simulink model "Sullivan_HodgkinHuxleyFinal"  (R2017a)
settings: Solver=ode45  StartTime=0.0  StopTime=100  RelTol=1e-3  EnableMultiTasking=on
settings Model: Creator=Andrew  LastModifiedBy=atsullivan
settings DataIOCC: LimitDataPoints=on  SaveFormat=Array
settings OptimizationCC: LifeSpan=inf
settings DebuggingCC: SFUnexpectedBacktrackingDiag=warning  SFNoUnconditionalDefaultTransitionDiag=warning  SFExecutionAtInitializationDiag=none
settings HardwareCC: ProdBitPerPointer=32  ProdBitPerSizeT=32  ProdBitPerPtrDiffT=32  ProdLargestAtomicFloat=None  ProdIntDivRoundTo=Undefined  ProdEndianess=Unspecified  ProdWordSize=32  ProdHWDeviceType=32-bit Generic
settings ModelReferenceCC: PropagateSignalLabelsOutOfModel=off
settings GRTTargetCC: TargetLangStandard=C89/C90 (ANSI)  GeneratePreprocessorConditionals=Disable all
settings ConfigComp: CovMetricSettings=dw  CovHtmlReporting=on  CovSaveCumulativeToWorkspaceVar=on  CovSaveSingleToWorkspaceVar=on  CovExternalEMLEnable=off

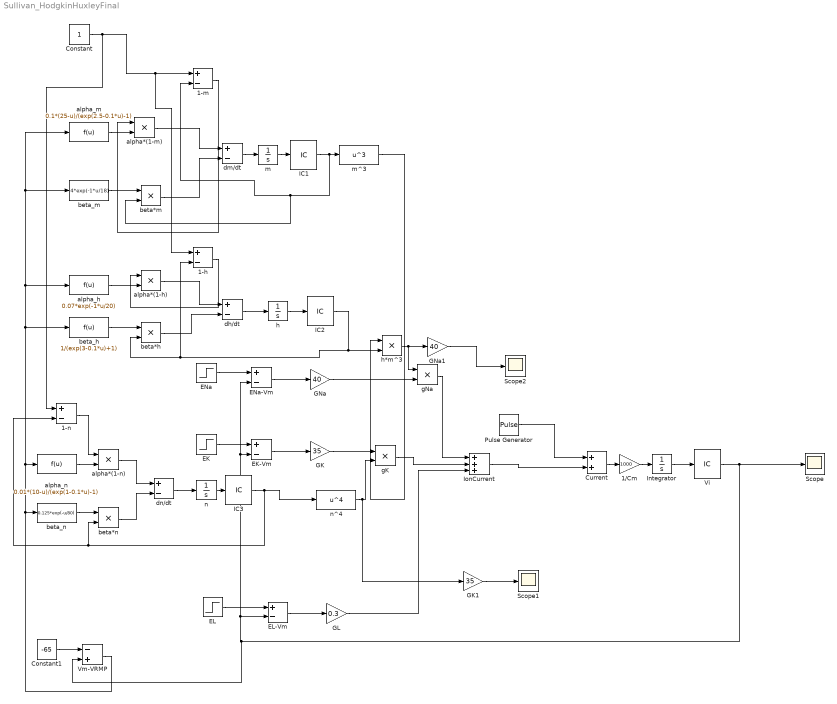
== system Sullivan_HodgkinHuxleyFinal ==
  1-h : Sum  Inputs=+-
  1-m : Sum  Inputs=+-
  1-n : Sum  Inputs=+-
  1/Cm : Gain  Gain=1000
  Constant : Constant
  Constant1 : Constant  Value=-65
  Current : Sum
  EK : Step  Before=-77  After=-77  SampleTime=0
  EK-Vm : Sum  Inputs=+-
  EL : Step  Before=-65  After=-65  SampleTime=0
  EL-Vm : Sum  Inputs=+-
  ENa : Step  Before=55  After=55  SampleTime=0
  ENa-Vm : Sum  Inputs=+-
  GK : Gain  Gain=35
  GK1 : Gain  Gain=35
  GL : Gain  Gain=0.3
  GNa : Gain  Gain=40
  GNa1 : Gain  Gain=40
  IC1 : InitialCondition  Value=0.0207
  IC2 : InitialCondition  Value=0.8194
  IC3 : InitialCondition  Value=0.3520
  Integrator : Integrator
  IonCurrent : Sum  Inputs=+++
  Pulse Generator : DiscretePulseGenerator  PulseType=Time based  Amplitude=20  Period=30  PulseWidth=10/3  PhaseDelay=30
  Scope : Scope
  Scope1 : Scope
  Scope2 : Scope
  Vi : InitialCondition  Value=-65
  Vm-VRMP : Sum  Inputs=-+
  alpha*(1-h) : Product
  alpha*(1-m) : Product
  alpha*(1-n) : Product
  alpha_h : Fcn  Expr=0.07*exp(-1*u/20)
  alpha_m : Fcn  Expr=0.1*(25-u)/(exp(2.5-0.1*u)-1)
  alpha_n : Fcn  Expr=0.01*(10-u)/(exp(1-0.1*u)-1)
  beta*h : Product
  beta*m : Product
  beta*n : Product
  beta_h : Fcn  Expr=1/(exp(3-0.1*u)+1)
  beta_m : Fcn  Expr=4*exp(-1*u/18)
  beta_n : Fcn  Expr=0.125*exp(-u/80)
  dh/dt : Sum  Inputs=+-
  dm/dt : Sum  Inputs=+-
  dn/dt : Sum  Inputs=+-
  gK : Product
  gNa : Product
  h : Integrator
  h*m^3 : Product
  m : Integrator
  m^3 : Fcn  Expr=u^3
  n : Integrator
  n^4 : Fcn  Expr=u^4
  wires:
  EL/1 -> EL-Vm/1
  EL-Vm/1 -> GL/1
  ENa-Vm/1 -> GNa/1
  ENa/1 -> ENa-Vm/1
  EK/1 -> EK-Vm/1
  GNa/1 -> gNa/2
  GK/1 -> gK/1
  gNa/1 -> IonCurrent/1
  gK/1 -> IonCurrent/2
  h*m^3/1 -> gNa/1, GNa1/1
  1/Cm/1 -> Integrator/1
  GL/1 -> IonCurrent/3
  Current/1 -> 1/Cm/1
  IonCurrent/1 -> Current/2
  Pulse Generator/1 -> Current/1
  Integrator/1 -> Vi/1
  m^3/1 -> h*m^3/1
  dm/dt/1 -> m/1
  alpha_m/1 -> alpha*(1-m)/2
  beta_m/1 -> beta*m/1
  Constant/1 -> 1-n/1, 1-h/1, 1-m/1
  1-m/1 -> alpha*(1-m)/1
  alpha*(1-m)/1 -> dm/dt/1
  beta*m/1 -> dm/dt/2
  dh/dt/1 -> h/1
  h/1 -> IC2/1
  beta_h/1 -> beta*h/1
  alpha_h/1 -> alpha*(1-h)/2
  beta*h/1 -> dh/dt/2
  1-h/1 -> alpha*(1-h)/1
  alpha*(1-h)/1 -> dh/dt/1
  alpha_n/1 -> alpha*(1-n)/2
  beta_n/1 -> beta*n/1
  1-n/1 -> alpha*(1-n)/1
  dn/dt/1 -> n/1
  alpha*(1-n)/1 -> dn/dt/1
  beta*n/1 -> dn/dt/2
  n^4/1 -> GK1/1, gK/2
  n/1 -> IC3/1
  EK-Vm/1 -> GK/1
  Constant1/1 -> Vm-VRMP/1
  Vm-VRMP/1 -> alpha_m/1, beta_m/1, alpha_h/1, beta_h/1, alpha_n/1, beta_n/1
  Vi/1 -> Vm-VRMP/2, ENa-Vm/2, EK-Vm/2, EL-Vm/2, Scope/1
  m/1 -> IC1/1
  IC1/1 -> 1-m/2, beta*m/2, m^3/1
  IC2/1 -> 1-h/2, beta*h/2, h*m^3/2
  IC3/1 -> 1-n/2, beta*n/2, n^4/1
  GNa1/1 -> Scope2/1
  GK1/1 -> Scope1/1
